simulink model "sl_groundvehicleDynamics"  (R2025b)
settings: Solver=ode45  StartTime=0.0  StopTime=1000  RelTol=1e-5  EnableMultiTasking=on
InitFcn:
  | mdl_robot;
undefined symbols (not defined in the file or in its folder): robot
libraries: simulink x5, mobileRoboticsLib x4, simulink_extras x4
settings Model: Creator=sriramn  LastModifiedBy=platt
settings SolverCC: ZeroCrossAlgorithm=Adaptive  AlgebraicLoopSolver=TrustRegion
settings DataIOCC: LimitDataPoints=on  SaveFormat=Array  ReturnWorkspaceOutputs=off
settings OptimizationCC: ReuseModelBlockBuffer=off  LifeSpan=inf
settings DebuggingCC: UnderspecifiedInitializationDetection=Classic  MergeDetectMultiDrivingBlocksExec=none  SolverPrmCheckMsg=warning  UnderSpecifiedDataTypeMsg=warning  UnconnectedInputMsg=warning  UnconnectedOutputMsg=warning  UnconnectedLineMsg=warning  AllowSymbolicDim=off  SFUnexpectedBacktrackingDiag=warning  SFNoUnconditionalDefaultTransitionDiag=warning  SFExecutionAtInitializationDiag=none  ArithmeticOperatorsInVariantConditions=warning
settings HardwareCC: ProdBitPerPointer=32.0  ProdBitPerSizeT=32.0  ProdBitPerPtrDiffT=32.0  ProdLargestAtomicFloat=None  ProdIntDivRoundTo=Undefined  ProdEndianess=Unspecified  ProdWordSize=32.0  ProdHWDeviceType=32-bit Generic
settings ModelReferenceCC: EnableRefExpFcnMdlSchedulingChecks=on  ModelReferenceMinAlgLoopOccurrences=on  PropagateSignalLabelsOutOfModel=off
settings SFSimCC: SimUseLocalCustomCode=off  CustomCodeUndefinedFunction=UseInterfaceOnly
settings RTWCC: RTWUseLocalCustomCode=off  GPUComputeCapability=3.5
settings CodeAppCC: StateflowObjectComments=on
settings GRTTargetCC: TargetLangStandard=C89/C90 (ANSI)
settings ConfigComp: CovMetricSettings=dw  CovSaveCumulativeToWorkspaceVar=on  CovSaveSingleToWorkspaceVar=on  CovExternalEMLEnable=off  CovSFcnEnable=off  PLC_RTWMaxIdLength=31.0  PLC_RemoveUnusedSSMethodCallArguments=off  PLC_InlineEnumCastFunction=off  PLC_ActiveTab=0.0  PLC_FoldFBCallOutputVar=off  PLC_TargetIDE=codesys35  PLC_MultiTBSigbuilderTimeRange=off  PLC_EnableUnsignedAndDoubleTypes=off  PLC_RollThreshold=5.0  PLC_Enable64bitIntSupport=off  PLC_MaxFieldsInUDT=500.0  PLC_UseCallOutputArgSyntax=off  PLC_EnableUDTSplitting=off  PLC_EnableStringLiteralTB=on
settings SimscapeCC: SimscapeNormalizeSystem=off
settings ConfigurationSet: Description=SimMechanics 2G
settings ExplorerConfigSet: InternalSimMechanicsExplorerSettings="<ExplorerConfiguration><canonicalview>planar_xy</canonicalview><AnimationSetting><BasePlaybackSpeed>1.0</BasePlaybackSpeed><PlaybackSpeedFactor>1.0</PlaybackSpeedFactor></AnimationSetting><TilePanel><TileInfo><Tiles Columns=\"1\" Count=\"1\" Rows=\"1\"><Column Left=\"2\" Weight=\"1\"/><Column Left=\"1628\"/><Row Top=\"2\" Weight=\"1\"/><Row Top=\"1072\"/><Tile Height=\"1\" Width=\"1\" X=\"0\" Y=\"0\"/></Tiles></TileInfo><SceneInfo><SceneViewer><BGColor><R>0.60000002384185791</R><G>0.60000002384185791</G><B>0.60000002384185791</B></BGColor><Camera><Position><X>0.22951840878551699</X><Y>0.32651610611526627</Y><Z>-0.27215421354393321</Z></Position><Center><X>-0.15775714411666431</X><Y>-0.15462825985839526</Y><Z>0.065702552916005602</Z></Center><Up><X>-0.56030137557930915</X><Y>0.72817587161684794</Y><Z>0.39474329445726858</Z></Up><Left>-0.21481383955700509</Left><Right>0.21481383955700509</Right><Bottom>-0.27569784609469139</Bottom><Top>0.27569784609469139</Top></Camera></SceneViewer></SceneInfo></TilePanel></ExplorerConfiguration>"

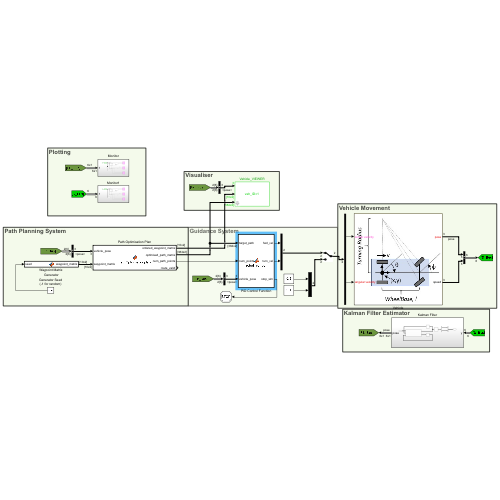
[thumbnail: Simulink's stored preview of the top-level diagram]
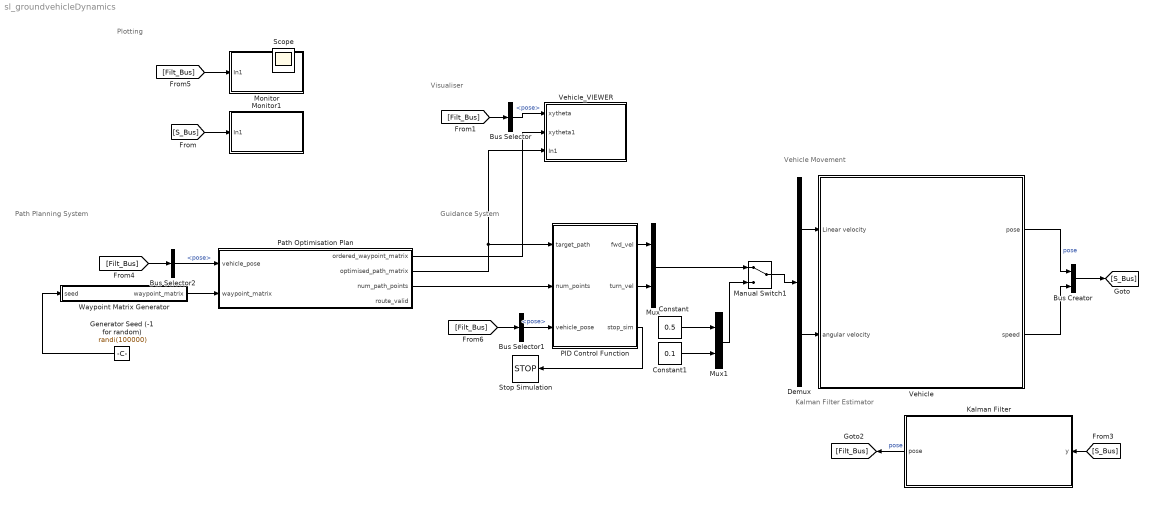
== system sl_groundvehicleDynamics ==
  note: Kalman Filter Estimator
  note: Plotting
  note: Vehicle Movement
  note: Guidance System
  note: Path Planning System
  note: Visualiser
  Bus Creator : BusCreator  Inputs=2
  Bus Selector : BusSelector  OutputSignals=pose
  Bus Selector1 : BusSelector  OutputSignals=pose
  Bus Selector2 : BusSelector  OutputSignals=pose
  Constant : Constant  Value=0.5
  Constant1 : Constant  Value=0.1
  Demux : Demux  Outputs=2
  Generator Seed (-1 for random) : Constant  Value=randi(100000)
  Kalman Filter : Subsystem
  Manual Switch1 : ManualSwitch
  Monitor : Subsystem
  Monitor1 : Subsystem
  Mux : Mux  Inputs=2
  Mux1 : Mux  Inputs=2
  PID Control Function : MATLAB Function  TreatAsAtomicUnit=on
  Path Optimisation Plan : MATLAB Function  TreatAsAtomicUnit=on
  Stop Simulation : Stop
  Vehicle : Subsystem
      mask Display: image('vehicle.jpg');
  Vehicle_VIEWER : Subsystem  mask{wp_mat=0, veh_init_xytheta=[robot.X robot.Y robot.Theta], veh_ID_num=1, Ts=0.5}
      mask prompts: wp_mat "Waypoint matrix for arena [x_col, y_col] (m)"; veh_init_xytheta "Initial pose [x,y,theta]"; veh_ID_num "Vehicle ID number"; Ts "Sample time for updating animation (secs)"
      mask TypeOptions veh_ID_num: 1 | 2 | 3 | 4
      mask DialogControl Control2 Prompt: Animate simulation of Differential Drive Robot (DDR)
      mask Display: fprintf('veh_ID=%d',veh_ID_num);
  Waypoint Matrix Generator : MATLAB Function  TreatAsAtomicUnit=on
  Scope : Scope
      settings: ActiveDisplayYMinimum=0.07  ActiveDisplayYMaximum=0.09
  wires:
  Generator Seed (-1 for random)/1 -> Waypoint Matrix Generator/1(seed)
  Waypoint Matrix Generator/1(waypoint_matrix) -> Path Optimisation Plan/2(waypoint_matrix)
  Bus Selector1/1 -> PID Control Function/3(vehicle_pose)  "<pose>"
  [Filt_Bus] -> Bus Selector2/1
  Bus Selector2/1 -> Path Optimisation Plan/1(vehicle_pose)  "<pose>"
  Bus Selector/1 -> Vehicle_VIEWER/1(xytheta)  "<pose>"
  [S_Bus] -> Monitor1/1(In1)
  [Filt_Bus] -> Monitor/1(In1)
  Vehicle/1(pose) -> Bus Creator/1  "pose"
  Vehicle/2(speed) -> Bus Creator/2
  [Filt_Bus] -> Bus Selector/1
  [S_Bus] -> Kalman Filter/1(y)
  [Filt_Bus] -> Bus Selector1/1
  Kalman Filter/1(pose) -> [Filt_Bus]  "pose"
  Bus Creator/1 -> [S_Bus]
  Path Optimisation Plan/2(optimised_path_matrix) -> Vehicle_VIEWER/3(In1), PID Control Function/1(target_path)
  PID Control Function/3(stop_sim) -> Stop Simulation/1
  Path Optimisation Plan/3(num_path_points) -> PID Control Function/2(num_points)
  Path Optimisation Plan/1(ordered_waypoint_matrix) -> Vehicle_VIEWER/2(xytheta1)
  Manual Switch1/1 -> Demux/1
  Constant/1 -> Mux1/1
  Mux1/1 -> Manual Switch1/2
  PID Control Function/1(fwd_vel) -> Mux/1
  PID Control Function/2(turn_vel) -> Mux/2
  Demux/2 -> Vehicle/2(angular velocity)
  Demux/1 -> Vehicle/1(Linear velocity)
  Constant1/1 -> Mux1/2
  Mux/1 -> Manual Switch1/1

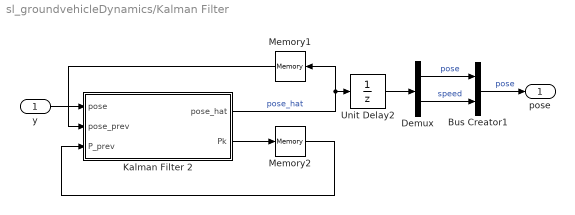
== system sl_groundvehicleDynamics/Kalman Filter ==
  y : Inport
  Bus Creator1 : BusCreator  Inputs=2
  Demux : Demux  Outputs=2
  Kalman Filter 2 : MATLAB Function  TreatAsAtomicUnit=on
  Memory1 : Memory  InheritSampleTime=on
  Memory2 : Memory  InheritSampleTime=on
  Unit Delay2 : UnitDelay  SampleTime=-1  HasFrameUpgradeWarning=on
  pose : Outport
  wires:
  Memory1/1 -> Kalman Filter 2/2(pose_prev)
  Kalman Filter 2/2(Pk) -> Memory2/1
  Kalman Filter 2/1(pose_hat) -> Unit Delay2/1, Memory1/1  "pose_hat"
  Memory2/1 -> Kalman Filter 2/3(P_prev)
  Demux/1 -> Bus Creator1/1  "pose"
  Bus Creator1/1 -> pose/1  "pose"
  Demux/2 -> Bus Creator1/2  "speed"
  y/1 -> Kalman Filter 2/1(pose)
  Unit Delay2/1 -> Demux/1

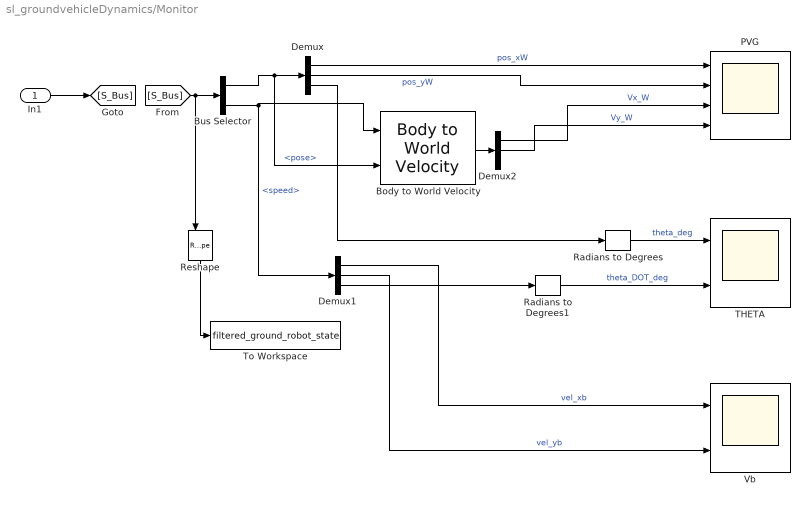
== system sl_groundvehicleDynamics/Monitor ==
  In1 : Inport
  Body to World Velocity : mobileRoboticsLib/Utilities/Body to World Velocity
      settings: SourceProductName=Mobile Robotics Simulation Toolbox
  Bus Selector : BusSelector  OutputSignals=pose,speed
  Demux : Demux  Outputs=3
  Demux1 : Demux  Outputs=3
  Demux2 : Demux  Outputs=3
  PVG : Scope  NumInputPorts=4
      settings: ActiveDisplayYMinimum=-3.02358  ActiveDisplayYMaximum=27.35477
  Radians to Degrees : simulink_extras/Transformations/Radians to Degrees
  Radians to Degrees1 : simulink_extras/Transformations/Radians to Degrees
  Reshape : Reshape  OutputDimensionality=Derive from reference input port
  THETA : Scope  NumInputPorts=2
      settings: ActiveDisplayYMinimum=-8.72937  ActiveDisplayYMaximum=60.06611  DataLoggingVariableName=ScopeData2
  To Workspace : ToWorkspace  VariableName=filtered_ground_robot_state  SampleTime=-1
  Vb : Scope  NumInputPorts=2
      settings: ActiveDisplayYMinimum=0.05577  ActiveDisplayYMaximum=0.8929
  wires:
  In1/1 -> [S_Bus]
  Demux/1 -> PVG/1  "pos_xW"
  Demux/2 -> PVG/2  "pos_yW"
  Radians to Degrees1/1 -> THETA/2  "theta_DOT_deg"
  Radians to Degrees/1 -> THETA/1  "theta_deg"
  Demux1/3 -> Radians to Degrees1/1
  Demux/3 -> Radians to Degrees/1
  Bus Selector/1 -> Body to World Velocity/2, Demux/1  "<pose>"
  Bus Selector/2 -> Demux1/1, Body to World Velocity/1  "<speed>"
  Body to World Velocity/1 -> Demux2/1
  Demux2/1 -> PVG/3  "Vx_W"
  Demux2/2 -> PVG/4  "Vy_W"
  Demux1/1 -> Vb/1  "vel_xb"
  Demux1/2 -> Vb/2  "vel_yb"
  [S_Bus] -> Bus Selector/1, Reshape/1
  Reshape/1 -> To Workspace/1

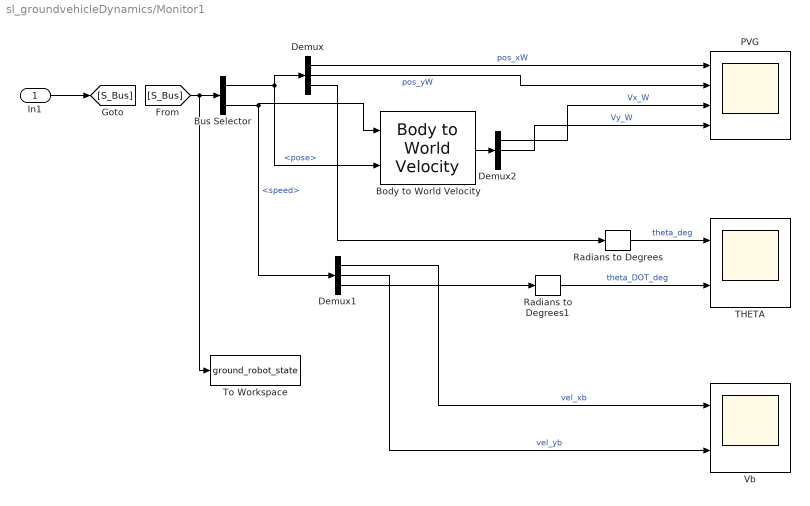
== system sl_groundvehicleDynamics/Monitor1 ==
  In1 : Inport
  Body to World Velocity : mobileRoboticsLib/Utilities/Body to World Velocity
      settings: SourceProductName=Mobile Robotics Simulation Toolbox
  Bus Selector : BusSelector  OutputSignals=pose,speed
  Demux : Demux  Outputs=3
  Demux1 : Demux  Outputs=3
  Demux2 : Demux  Outputs=3
  PVG : Scope  NumInputPorts=4
      settings: ActiveDisplayYMinimum=-3.02358  ActiveDisplayYMaximum=27.35477
  Radians to Degrees : simulink_extras/Transformations/Radians to Degrees
  Radians to Degrees1 : simulink_extras/Transformations/Radians to Degrees
  THETA : Scope  NumInputPorts=2
      settings: ActiveDisplayYMinimum=-8.72937  ActiveDisplayYMaximum=60.06611  DataLoggingVariableName=ScopeData2
  To Workspace : ToWorkspace  VariableName=ground_robot_state  SampleTime=-1
  Vb : Scope  NumInputPorts=2
      settings: ActiveDisplayYMinimum=0.05577  ActiveDisplayYMaximum=0.8929
  wires:
  In1/1 -> [S_Bus]
  [S_Bus] -> To Workspace/1, Bus Selector/1
  Demux/1 -> PVG/1  "pos_xW"
  Demux/2 -> PVG/2  "pos_yW"
  Radians to Degrees1/1 -> THETA/2  "theta_DOT_deg"
  Radians to Degrees/1 -> THETA/1  "theta_deg"
  Demux1/3 -> Radians to Degrees1/1
  Demux/3 -> Radians to Degrees/1
  Bus Selector/1 -> Body to World Velocity/2, Demux/1  "<pose>"
  Body to World Velocity/1 -> Demux2/1
  Demux2/1 -> PVG/3  "Vx_W"
  Demux2/2 -> PVG/4  "Vy_W"
  Demux1/1 -> Vb/1  "vel_xb"
  Demux1/2 -> Vb/2  "vel_yb"
  Bus Selector/2 -> Demux1/1, Body to World Velocity/1  "<speed>"

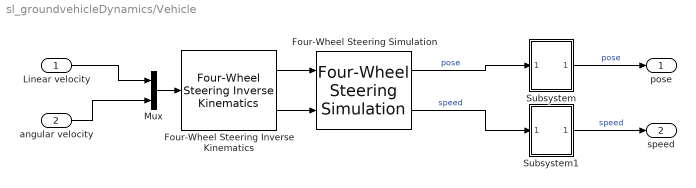
== system sl_groundvehicleDynamics/Vehicle ==
  Linear velocity : Inport
  angular velocity : Inport  Port=2
  Four-Wheel Steering Inverse Kinematics : mobileRoboticsLib/Kinematic Models/Four-Wheel Steering/Four-Wheel Steering Inverse Kinematics  wheelRadius=0.1  frontWheelDist=0.25  rearWheelDist=0.25  ikMode=Front Steering
      settings: SourceProductName=Mobile Robotics Simulation Toolbox
  Four-Wheel Steering Simulation : mobileRoboticsLib/Kinematic Models/Four-Wheel Steering/Four-Wheel Steering Simulation  wheelRadius=0.1  frontWheelDist=0.25  rearWheelDist=0.25  initX=robot.X  initY=robot.Y  initAngle=robot.Theta  Ts=0.05
      settings: SourceProductName=Mobile Robotics Simulation Toolbox
  Mux : Mux  Inputs=2
  Subsystem : Subsystem
  Subsystem1 : Subsystem
  pose : Outport  VectorParamsAs1DForOutWhenUnconnected=off
  speed : Outport  Port=2
  wires:
  angular velocity/1 -> Mux/2
  Linear velocity/1 -> Mux/1
  Mux/1 -> Four-Wheel Steering Inverse Kinematics/1
  Four-Wheel Steering Simulation/1 -> Subsystem/1(In1)  "pose"
  Four-Wheel Steering Simulation/2 -> Subsystem1/1(In1)  "speed"
  Four-Wheel Steering Inverse Kinematics/1 -> Four-Wheel Steering Simulation/1
  Four-Wheel Steering Inverse Kinematics/2 -> Four-Wheel Steering Simulation/2
  Subsystem/1(pose) -> pose/1  "pose"
  Subsystem1/1(speed) -> speed/1  "speed"

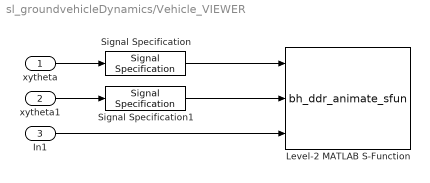
== system sl_groundvehicleDynamics/Vehicle_VIEWER ==
  xytheta : Inport
  xytheta1 : Inport  Port=2
  In1 : Inport  Port=3
  Level-2 MATLAB S-Function : M-S-Function  FunctionName=bh_ddr_animate_sfun  Parameters=Ts, wp_mat, veh_ID_num, veh_init_xytheta
  Signal Specification : SignalSpecification  Dimensions=3
  Signal Specification1 : SignalSpecification  Dimensions=[10 2]
  wires:
  xytheta/1 -> Signal Specification/1
  Signal Specification/1 -> Level-2 MATLAB S-Function/1
  xytheta1/1 -> Signal Specification1/1
  Signal Specification1/1 -> Level-2 MATLAB S-Function/2
  In1/1 -> Level-2 MATLAB S-Function/3

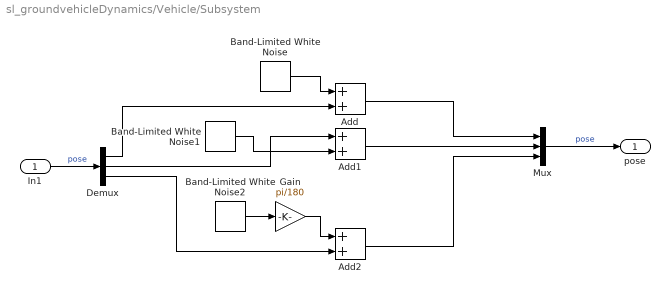
== system sl_groundvehicleDynamics/Vehicle/Subsystem ==
  In1 : Inport
  Add : Sum
  Add1 : Sum
  Add2 : Sum
  Band-Limited White Noise : simulink/Sources/Band-Limited White Noise  Cov=[0.001]  Ts=0.1  seed=[23341]
  Band-Limited White Noise1 : simulink/Sources/Band-Limited White Noise  Cov=[0.001]  Ts=0.1  seed=[10341]
  Band-Limited White Noise2 : simulink/Sources/Band-Limited White Noise  Cov=[0.41]  Ts=0.1  seed=[20341]
  Demux : Demux  Outputs=3
  Gain : Gain  Gain=pi/180
  Mux : Mux  Inputs=3
  pose : Outport
  wires:
  Add1/1 -> Mux/2
  Add2/1 -> Mux/3
  Demux/2 -> Add1/1
  Band-Limited White Noise2/1 -> Gain/1
  Demux/3 -> Add2/2
  Band-Limited White Noise/1 -> Add/1
  In1/1 -> Demux/1  "pose"
  Demux/1 -> Add/2
  Gain/1 -> Add2/1
  Mux/1 -> pose/1  "pose"
  Add/1 -> Mux/1
  Band-Limited White Noise1/1 -> Add1/2

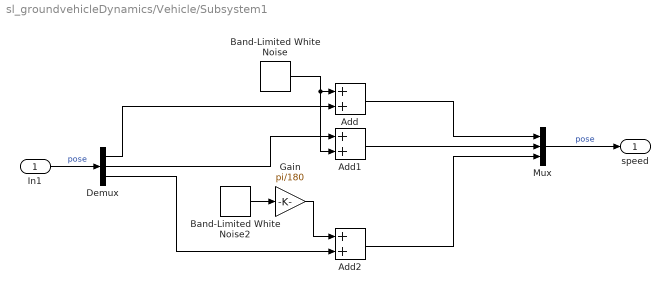
== system sl_groundvehicleDynamics/Vehicle/Subsystem1 ==
  In1 : Inport
  Add : Sum
  Add1 : Sum
  Add2 : Sum
  Band-Limited White Noise : simulink/Sources/Band-Limited White Noise  Cov=[0.001]  Ts=0.1  seed=[23341]
  Band-Limited White Noise2 : simulink/Sources/Band-Limited White Noise  Cov=[0.41]  Ts=0.1  seed=[23341]
  Demux : Demux  Outputs=3
  Gain : Gain  Gain=pi/180
  Mux : Mux  Inputs=3
  speed : Outport
  wires:
  Add1/1 -> Mux/2
  Add2/1 -> Mux/3
  Demux/2 -> Add1/1
  Band-Limited White Noise2/1 -> Gain/1
  Demux/3 -> Add2/2
  Band-Limited White Noise/1 -> Add1/2, Add/1
  In1/1 -> Demux/1  "pose"
  Demux/1 -> Add/2
  Gain/1 -> Add2/1
  Mux/1 -> speed/1  "pose"
  Add/1 -> Mux/1

== matlab function sl_groundvehicleDynamics/Kalman Filter/Kalman Filter 2 ==
  data: pose_hat output double size=[6 1] [0..50]; pose input size=6 [0..50]; pose_prev input [0..50]; Pk output size=[6 6]; P_prev input
function [pose_hat, Pk] = kalman_filter(pose, pose_prev, P_prev)
% KALMAN_FILTER
% 6-state Kalman filter for estimating robot pose and velocity.
%
% State vector:
%   x = [x; y; theta; x_dot; y_dot; theta_dot]
%
% Inputs:
%   pose      - measured state [x; y; theta; x_dot; y_dot; theta_dot]
%   pose_prev - previous estimated state
%   P_prev    - previous covariance matrix
%
% Outputs:
%   pose_hat  - estimated state [x; y; theta; x_dot; y_dot; theta_dot]
%   Pk        - updated covariance matrix

% -------------------------------------------------------------------------
% PERSISTENT VARIABLES
persistent first_entry
persistent counter

% Initialise persistent variables on first execution
if isempty(first_entry)
    first_entry = true;
end

if isempty(counter)
    counter = 0;
end

% -------------------------------------------------------------------------
% INITIAL STATE
% State: [x; y; theta; x_dot; y_dot; theta_dot]

% x0 = [robot.X; robot.Y; robot.Theta; 0; 0; 0];

% -------------------------------------------------------------------------
% KALMAN FILTER PARAMETERS
dt = 0.05; % Sampling time

% Process noise
sigma_pos = 0.1; % metres^2
sigma_theta = 2 * (pi/180)^2;
sigma_v = 2 * sigma_pos / dt^2;        % = 2*0.1/0.05^2 = 80 (m/s)^2
sigma_omega = 2 * sigma_theta / dt^2;  % = 2*(2*(pi/180)^2)/0.05^2 ≈ 0.244 (rad/s)^2

R = diag([sigma_pos, sigma_pos, sigma_theta, ...
          0.1, 0.1, sigma_theta]); % Measurement noise

% -------------------------------------------------------------------------
% STATE TRANSITION MATRIX

% Constant velocity model:
%
% x(k+1)     = x(k)     + x_dot(k)*dt
% y(k+1)     = y(k)     + y_dot(k)*dt
% theta(k+1) = theta(k) + theta_dot(k)*dt

A = [1  0  0  dt 0  0;
     0  1  0  0  dt 0;
     0  0  1  0  0  dt;
     0  0  0  1  0  0;
     0  0  0  0  1  0;
     0  0  0  0  0  1];

% -------------------------------------------------------------------------
% MEASUREMENT MATRIX
% All states are measured
H = [1 0 0 0 0 0;
     0 1 0 0 0 0;
     0 0 1 0 0 0;
     0 0 0 1 0 0;
     0 0 0 0 1 0;
     0 0 0 0 0 1];

% -------------------------------------------------------------------------
% PROCESS NOISE COVARIANCE
Q = diag([ ...
    sigma_pos/10, ...
    sigma_pos/10, ...
    sigma_theta/500, ...
    sigma_pos/100, ...
    sigma_pos/10000000000, ...
    sigma_theta/100]);

% -------------------------------------------------------------------------
% INITIALISE FILTER
if first_entry
    xkh = pose; % Initialise state from the first measured pose.
    xkh(1:6) = pose(1:6);
    xkh(5) = 0; 
    Pk = diag([1, 1, 1, 1, 0, 1]); % Large initial covariance means the initial estimate is uncertain.
else
    % Use the previous estimated state and covariance.
    xkh = pose_prev;
    Pk  = P_prev;
end

% -------------------------------------------------------------------------
% PREDICTION STEP
x_pred = A * xkh; % Predict the next state using the motion model.
% x_pred(3) = wrapToPi(x_pred(3));
P_pred = A * Pk * A' + Q; % Predict the covariance.

% -------------------------------------------------------------------------
% MEASUREMENT UPDATE
innovation = pose(1:6) - H * x_pred; % Measurement residual / innovation.

% innovation(3) = wrapToPi(innovation(3)); % Prevent heading angle discontinuity.

S = H * P_pred * H' + R; % Innovation covariance.

K = P_pred * H' / S; % Kalman gain.

xkh = x_pred + K * innovation; % Correct predicted state using measurement.

% xkh(3) = wrapToPi(xkh(3)); % Ensure heading remains within [-pi, pi].

Pk = (eye(6) - K * H) * P_pred; % Update covariance.

% -------------------------------------------------------------------------
% OUTPUT
pose_hat = xkh;

% -------------------------------------------------------------------------
% UPDATE FILTER STATUS
counter = counter + 1;
first_entry = false;

end

== matlab function sl_groundvehicleDynamics/PID Control Function ==
  data: target_path input; num_points input; vehicle_pose input; fwd_vel output size=1; turn_vel output size=1; stop_sim output
function [fwd_vel, turn_vel, stop_sim] = robot_control(target_path, num_points, vehicle_pose)
%% Tuning Parameters
look_ahead_dis = 3.0;
waypoint_threshold = 0.4;
end_dist = 0.25;

% cap top speed and turn velocity
top_speed=5;
max_omega=deg2rad(12);

% Gains
Krho = 0.6; % speed based on distance 
Ktheta = 0.50;
Kd = 2.7;
Ki = 0.01; 

%% Initial waypoint index and error values
persistent waypoint_index; 
persistent om_err_prev;
persistent stop;

if isempty(waypoint_index)
    waypoint_index=1; % first waypoint
    om_err_prev=0;
    stop=0;
end

%% Extract current pose and target path (once)
persistent x_goals;
persistent y_goals;
persistent num_valid_points;

if isempty(x_goals)
    x_goals=target_path(1:num_points,1);
    y_goals=target_path(1:num_points,2);
    num_valid_points=num_points;
end

x_pos=vehicle_pose(1); y_pos=vehicle_pose(2); theta_ori=vehicle_pose(3);

%% RVWP

% Distance to current waypoint
Ru = sqrt((x_pos - x_goals(waypoint_index))^2 + ...
           (y_pos - y_goals(waypoint_index))^2);
% Distance to next waypoint
waypoint_dist = sqrt((x_pos - x_goals(waypoint_index+1))^2 + ...
                     (y_pos - y_goals(waypoint_index+1))^2);

% Desired path direction (path vector)
path_vec_x = x_goals(waypoint_index+1) - x_goals(waypoint_index);
path_vec_y = y_goals(waypoint_index+1) - y_goals(waypoint_index);
theta_target = atan2(path_vec_y, path_vec_x);

% Angle from vehicle orientation to current waypoint
to_bot_x = x_pos - x_goals(waypoint_index);
to_bot_y = y_pos - y_goals(waypoint_index);
theta_to_waypoint = atan2(to_bot_y, to_bot_x);

% Angle difference
beta = angdiff(theta_to_waypoint, theta_target);

% Distance along desired path
R = sqrt(Ru^2 - (Ru*sin(beta))^2);

% Receding Vector WayPoint using look ahead distance
x_star = x_goals(waypoint_index) + (R + look_ahead_dis)*cos(theta_target);
y_star = y_goals(waypoint_index) + (R + look_ahead_dis)*sin(theta_target);

%% Run Control Law
diff_x = x_star - x_pos;
diff_y = y_star - y_pos;
rho = sqrt(diff_x^2 + diff_y ^2);
gamma = atan2(diff_y,diff_x);

alpha = angdiff(theta_ori, gamma); 

% proportional control for velocity
vel = Krho*rho*cos(alpha);

% pid control for angular velocity
om_err = angdiff(theta_ori, gamma);
om_err_dot = (om_err_prev-om_err);
om_int = om_err_prev + om_err;

omega = Ktheta*om_err + Kd*om_err_dot + Ki*om_int;
om_err_prev=om_err;

%% Near Condition for Waypoint Progression
if (waypoint_dist < waypoint_threshold) ...
    && (waypoint_index < num_valid_points-1)
    waypoint_index=waypoint_index+1;
end

% Additional check for overshoot detection
if waypoint_index < num_valid_points-1
    dot_prod = path_vec_x*to_bot_x + path_vec_y*to_bot_y;
    path_len_sq = path_vec_x^2 + path_vec_y^2;

    if dot_prod > path_len_sq
        waypoint_index=waypoint_index+1;
    end
end

%% End Sim
if waypoint_index >= num_valid_points-1
    dist_to_final_wp = sqrt((x_pos - x_goals(end))^2 ...
                          + (y_pos - y_goals(end))^2);
    if dist_to_final_wp < end_dist
        stop=1;
    end
end

%% Output Capped Vehicle Commands
vel = max(min(vel, top_speed), -top_speed);
omega = max(min(omega, max_omega), -max_omega);

fwd_vel=vel;
turn_vel=omega;
stop_sim=stop;

== matlab function sl_groundvehicleDynamics/Waypoint Matrix Generator ==
  data: seed input; waypoint_matrix output
function waypoint_matrix = fcn(seed)

    % Define coordinate bounds
    coordMin = -100;
    coordMax = 100;
    numPoints = 10;

    persistent waypoints
    if isempty(waypoints)
        % Seed the generator only if a valid (non-negative) seed is given
        % If seed < 0 (ie -1) then default random state is used
        if seed >= 0
            rng(seed);
        end

        % Generate random integer coordinates within bounds
        waypoints = randi([coordMin coordMax], numPoints, 2);
    end
    waypoint_matrix=waypoints;
end

== matlab function sl_groundvehicleDynamics/Path Optimisation Plan ==
  data: ordered_waypoint_matrix output; optimised_path_matrix output; num_path_points output; route_valid output; vehicle_pose input; waypoint_matrix input
function [ordered_waypoint_matrix, optimised_path_matrix, num_path_points, route_valid] = PathOptimisationplan(vehicle_pose, waypoint_matrix)
%#codegen
% Version: Design B group handoff, 2026-08-22.
% Role: overhead path optimiser and dense-route generator.
% Overhead planner/cache.
% Orders the waypoints once, generates a dense route once, and outputs the
% dense route for Matt's guidance/control block.

% Number of mission waypoints expected from the waypoint generator.
NUM_WAYPOINTS = 10;

% Fixed route-buffer capacity. This must match the PID block cache size.
% Increase this if smaller PATH_SPACING values create more dense points.
MAX_ROUTE_POINTS = 384;

% Desired distance between generated dense path points, in metres.
% Smaller spacing gives smoother guidance but consumes more route-buffer rows.
PATH_SPACING = 5.0;

persistent orderedWaypoints routePath routePoints routeReady lastWaypointMatrix

if isempty(routeReady)
    orderedWaypoints = zeros(NUM_WAYPOINTS, 2);
    routePath = zeros(MAX_ROUTE_POINTS, 2);
    routePoints = 0;
    routeReady = 0;
    lastWaypointMatrix = zeros(NUM_WAYPOINTS, 2);
end

ordered_waypoint_matrix = orderedWaypoints;
optimised_path_matrix = routePath;
num_path_points = routePoints;
route_valid = routeReady;

if ~hasValidInputs(vehicle_pose, waypoint_matrix)
    ordered_waypoint_matrix = zeros(NUM_WAYPOINTS, 2);
    optimised_path_matrix = zeros(MAX_ROUTE_POINTS, 2);
    num_path_points = 0;
    route_valid = 0;
    return;
end

x = vehicle_pose(1);
y = vehicle_pose(2);

if routeReady == 0 || waypointMatrixChanged(waypoint_matrix, lastWaypointMatrix)
    [orderedWaypoints, orderValid] = optimiseWaypointOrderHeldKarp(waypoint_matrix, x, y);
    [routePath, routePoints, denseValid] = buildDenseRoute([x, y], orderedWaypoints, PATH_SPACING, MAX_ROUTE_POINTS);
    routeReady = orderValid * denseValid;
    lastWaypointMatrix = waypoint_matrix;
end

ordered_waypoint_matrix = orderedWaypoints;
optimised_path_matrix = routePath;
num_path_points = routePoints;
route_valid = routeReady;
end

% Validate Simulink inputs before route generation.
function tf = hasValidInputs(vehicle_pose, waypoint_matrix)
tf = true;

if numel(vehicle_pose) < 3
    tf = false;
    return;
end

if size(waypoint_matrix, 1) < 10 || size(waypoint_matrix, 2) < 2
    tf = false;
    return;
end

if ~isfinite(vehicle_pose(1)) || ~isfinite(vehicle_pose(2)) || ~isfinite(vehicle_pose(3))
    tf = false;
    return;
end

for row = 1:10
    if ~isfinite(waypoint_matrix(row, 1)) || ~isfinite(waypoint_matrix(row, 2))
        tf = false;
        return;
    end
end
end

% Detect waypoint changes so the expensive optimiser only reruns when needed.
function changed = waypointMatrixChanged(currentMatrix, previousMatrix)
changed = false;

for row = 1:10
    for col = 1:2
        if abs(currentMatrix(row, col) - previousMatrix(row, col)) > 1e-9
            changed = true;
            return;
        end
    end
end
end

% Convert the optimised sparse waypoint order into a fixed-size dense route.
function [routePath, numRoutePoints, success] = buildDenseRoute(startPoint, orderedWaypoints, spacing, maxRoutePoints)
NUM_WAYPOINTS = 10;

routePath = zeros(maxRoutePoints, 2);
numRoutePoints = 1;
success = 1;
routePath(1, :) = startPoint;

previousPoint = startPoint;
spacing = max(spacing, 0.5);

for waypoint = 1:NUM_WAYPOINTS
    nextPoint = orderedWaypoints(waypoint, :);
    dx = nextPoint(1) - previousPoint(1);
    dy = nextPoint(2) - previousPoint(2);
    legLength = hypot(dx, dy);

    if legLength < 1e-9
        previousPoint = nextPoint;
        continue;
    end

    steps = max(1, ceil(legLength / spacing));
    for step = 1:steps
        if numRoutePoints >= maxRoutePoints
            success = 0;
            return;
        end

        alpha = step / steps;
        numRoutePoints = numRoutePoints + 1;
        routePath(numRoutePoints, :) = previousPoint + alpha * (nextPoint - previousPoint);
    end

    previousPoint = nextPoint;
end
end

% Build the waypoint cost matrix and return the optimal open-route order.
function [orderedWaypoints, success] = optimiseWaypointOrderHeldKarp(waypoint_matrix, vehicle_pos_x, vehicle_pos_y)
NUM_WAYPOINTS = 10;

orderedWaypoints = zeros(NUM_WAYPOINTS, 2);
success = 0;

points = zeros(NUM_WAYPOINTS + 1, 2);
points(1, :) = [vehicle_pos_x, vehicle_pos_y];

for waypoint = 1:NUM_WAYPOINTS
    points(waypoint + 1, :) = waypoint_matrix(waypoint, :);
end

costMatrix = zeros(NUM_WAYPOINTS + 1, NUM_WAYPOINTS + 1);

for row = 1:(NUM_WAYPOINTS + 1)
    for col = 1:(NUM_WAYPOINTS + 1)
        dx = points(row, 1) - points(col, 1);
        dy = points(row, 2) - points(col, 2);
        costMatrix(row, col) = hypot(dx, dy);
    end
end

[routeOrder, routeSuccess] = solveOpenTspHeldKarp(costMatrix);

if routeSuccess == 0
    return;
end

for waypoint = 1:NUM_WAYPOINTS
    orderedWaypoints(waypoint, :) = waypoint_matrix(routeOrder(waypoint), :);
end

success = 1;
end

% Solve the 10-waypoint open TSP exactly using Held-Karp dynamic programming.
function [routeOrder, success] = solveOpenTspHeldKarp(costMatrix)
NUM_WAYPOINTS = 10;

% 2^10 masks are required for all waypoint-visited subsets.
MAX_MASKS = 1024;

routeOrder = zeros(NUM_WAYPOINTS, 1);
success = 0;

dp = inf(MAX_MASKS, NUM_WAYPOINTS);
parent = zeros(MAX_MASKS, NUM_WAYPOINTS);

for waypoint = 1:NUM_WAYPOINTS
    mask = bitshift(1, waypoint - 1);
    dp(mask + 1, waypoint) = costMatrix(1, waypoint + 1);
end

fullMask = bitshift(1, NUM_WAYPOINTS) - 1;

for mask = 1:fullMask
    for lastWaypoint = 1:NUM_WAYPOINTS
        currentCost = dp(mask + 1, lastWaypoint);

        if ~isfinite(currentCost)
            continue;
        end

        for nextWaypoint = 1:NUM_WAYPOINTS
            nextBit = bitshift(1, nextWaypoint - 1);

            if bitand(mask, nextBit) ~= 0
                continue;
            end

            nextMask = bitor(mask, nextBit);
            candidateCost = currentCost + costMatrix(lastWaypoint + 1, nextWaypoint + 1);

            if candidateCost < dp(nextMask + 1, nextWaypoint)
                dp(nextMask + 1, nextWaypoint) = candidateCost;
                parent(nextMask + 1, nextWaypoint) = lastWaypoint;
            end
        end
    end
end

bestCost = inf;
lastBest = 0;

for lastWaypoint = 1:NUM_WAYPOINTS
    candidateCost = dp(fullMask + 1, lastWaypoint);
    if candidateCost < bestCost
        bestCost = candidateCost;
        lastBest = lastWaypoint;
    end
end

if lastBest == 0 || ~isfinite(bestCost)
    return;
end

mask = fullMask;
lastWaypoint = lastBest;

for position = NUM_WAYPOINTS:-1:1
    routeOrder(position) = lastWaypoint;
    previousWaypoint = parent(mask + 1, lastWaypoint);
    mask = mask - bitshift(1, lastWaypoint - 1);
    lastWaypoint = previousWaypoint;
end

success = 1;
end
